simulink model "Event5_2018a"  (R2018a)
settings: Solver=FixedStepDiscrete  StartTime=0.0  StopTime=0.1  FixedStep=0.1  RelTol=1e-3  EnableMultiTasking=on
settings Model: Creator=BEAR  LastModifiedBy=bzhan
settings SolverCC: AutoInsertRateTranBlk=on
settings DataIOCC: LimitDataPoints=on
settings OptimizationCC: LifeSpan=inf
settings DebuggingCC: AllowSymbolicDim=off  SFUnexpectedBacktrackingDiag=warning  SFNoUnconditionalDefaultTransitionDiag=warning  SFExecutionAtInitializationDiag=none
settings CodeAppCC: StateflowObjectComments=on
settings GRTTargetCC: TargetLangStandard=C89/C90 (ANSI)
settings ConfigComp: CovMetricSettings=dw  CovHtmlReporting=on  CovSaveCumulativeToWorkspaceVar=on  CovSaveSingleToWorkspaceVar=on  CovShowResultsExplorer=off  CovExternalEMLEnable=off  CovSFcnEnable=off

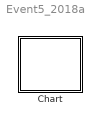
== system Event5_2018a ==
  Chart : Stateflow chart  TreatAsAtomicUnit=on

== stateflow chart Event5_2018a/Chart ==
  state A [parallel]
    settings: executionOrder=1
    state A1
    state A2
      en: f("en_A2")
    state A3
      en: f("en_A3")
    (default) -> A1 : {x=-1;}
    A1 -> A2
    A2 -> A3
  state B [parallel]
    settings: executionOrder=2
    state B1
    state B2
      en: f("en_B2")
    (default) -> B1
    B1 -> B2 : {f("b")}/{E;f("tb")}
  data: s function_input; x local
  events: E local FUNCTION_CALL_EVENT; F local FUNCTION_CALL_EVENT
  function f(s):
    | function f(s)
    |   fprintf(s+"\n");
